simulink model "thermal_closed_loop_model"  (R2023a)
settings: Solver=ode23t  StartTime=0.0  StopTime=600  RelTol=1e-3
PostLoadFcn:
  | run('thermal_model_parameters.m')
  | run('thermal_harness_parameters.m')
  | run('thermal_variants_config.m')
values from neighbouring files (symbols this model uses):
  air_cp = 1004    [cathode_subsystem_parameters.m]    (also in thermal_subsystem_parameters.m)
  air_HC_min = 10    [cathode_subsystem_parameters.m]    (also in thermal_subsystem_parameters.m)
  air_HC_nom = 100    [cathode_subsystem_parameters.m]    (also in thermal_subsystem_parameters.m)
  air_rho = 1.2    [cathode_subsystem_parameters.m]    (also in thermal_subsystem_parameters.m)
  air_vel_nom = 1    [cathode_subsystem_parameters.m]    (also in thermal_subsystem_parameters.m)
  coolant_initial_pressure = 0.111325    [cathode_subsystem_parameters.m]    (also in thermal_subsystem_parameters.m)
  coolant_initial_temperature = 293.15    [cathode_subsystem_parameters.m]    (also in thermal_subsystem_parameters.m)
  coolant_tube_D = 0.05    [cathode_subsystem_parameters.m]    (also in thermal_subsystem_parameters.m)
  Hydrowell_VTS =     [Hydrowell_values_VLV.mat]
  radiator_area_air = 0.10260000000000001    (= 0.1026)    [cathode_subsystem_parameters.m]    (also in thermal_subsystem_parameters.m)
  radiator_area_fins = 2.5436250000000005    (= 2.543625)    [cathode_subsystem_parameters.m]    (also in thermal_subsystem_parameters.m)
  radiator_area_primary = 0.44452500000000011    (= 0.444525)    [cathode_subsystem_parameters.m]    (also in thermal_subsystem_parameters.m = 2 * radiator_tube_length * radiator_width * (radiator_fin_ro)
  radiator_n_tubes = 20    [cathode_subsystem_parameters.m]    (also in thermal_subsystem_parameters.m)
  radiator_tube_height = 0.0015    [cathode_subsystem_parameters.m]    (also in thermal_subsystem_parameters.m)
  radiator_tube_length = 0.45    [cathode_subsystem_parameters.m]    (also in thermal_subsystem_parameters.m)
  radiator_width = 0.025    [cathode_subsystem_parameters.m]    (also in thermal_subsystem_parameters.m)
  tcp_time_constant = 2    [cathode_subsystem_parameters.m]    (also in thermal_subsystem_parameters.m)
undefined symbols (not defined in the file or in its folder): sigbuilder_block, stack
libraries: fl_lib x153, nesl_utility x122, SimscapeFluids_lib x16, slpidlib x5, simulink x1
(part 2 of 8)

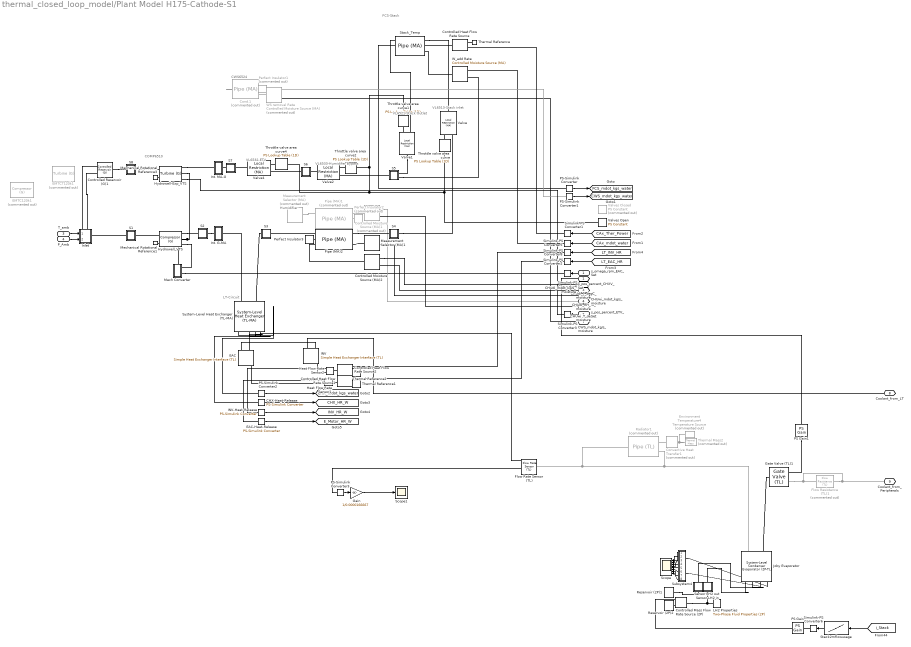
== system thermal_closed_loop_model/Plant Model H175-Cathode-S1 ==
  note: LT-Circuit
  note: Humidifier
  note: COMP6510
  note: FCS-Stack
  note: VL6513-Stack inlet
  note: VL6521-Stack Outlet
  note: VL6533-Humidifer Bypass
  note: CWS6524
  note: VL6532-ETV
  s_omega_rpm_EAC_Set : Inport
  s_pos_percent_ETV_Set : Inport  Port=2
  T_amb : Inport  Port=3
  P_Amb : Inport  Port=4
  CHX-Heat-Release : nesl_utility/PS-Simulink Converter  PhysicalDomain=network_engine_domain  SubClassName=ps_output  LeftPortType=input  RightPortType=output  PseudoPeriodic=off  Frequencies=[]  VectorFormat=inherit  Unit=inherit  AffineConversion=off
  Cond.1 : fl_lib/Moist Air/Elements/Pipe (MA)  Commented=on  length=1 m  area=1 m^2  Dh=.1 m  length_add=.1 m  roughness=15e-6 m  Re_lam=2000  Re_tur=4000  shape_factor=64  Nu_lam=3.66  wall_condensation=simscape.enum.onoff.on  RH_ws=.2  time_constant=1e-3 s  moisture_trace_gas_source=foundation.enum.moisture_trace_gas_source.controlled  moisture_source_spec=foundation.enum.moisture_source_spec.vapor  moisture_mass_flow=0 kg/s  moisture_temperature_spec=foundation.enum.temperature_spec.atmospheric  moisture_temperature=293.15 K  trace_gas_mass_flow=0 kg/s  trace_gas_temperature_spec=foundation.enum.temperature_spec.atmospheric  trace_gas_temperature=293.15 K  p_I_specify=off  p_I_priority=High  p_I=0.101325 MPa  p_I_nominal_specify=off  p_I_nominal_unit=MPa  p_I_nominal_value=1  T_I_specify=off  T_I_priority=High  T_I=293.15 K  T_I_nominal_specify=off  T_I_nominal_unit=K  T_I_nominal_value=1  RH_I_specify=off  RH_I_priority=High  RH_I=0  RH_I_nominal_specify=off  RH_I_nominal_unit=1  RH_I_nominal_value=1  x_w_I_specify=off  x_w_I_priority=None  x_w_I=0  x_w_I_nominal_specify=off  x_w_I_nominal_unit=1  x_w_I_nominal_value=1  y_w_I_specify=off  y_w_I_priority=None  y_w_I=0  y_w_I_nominal_specify=off  y_w_I_nominal_unit=1  y_w_I_nominal_value=1  HR_I_specify=off  HR_I_priority=None  HR_I=0  HR_I_nominal_specify=off  HR_I_nominal_unit=1  HR_I_nominal_value=1  x_g_I_specify=off  x_g_I_priority=High  x_g_I=0  x_g_I_nominal_specify=off  x_g_I_nominal_unit=1  x_g_I_nominal_value=1  y_g_I_specify=off  y_g_I_priority=None  y_g_I=0  y_g_I_nominal_specify=off  y_g_I_nominal_unit=1  y_g_I_nominal_value=1
      settings: InternalSimscapePortConfiguration="{\"Bottom\":[],\"Left\":[{\"id\":\"A\",\"label\":\"A\",\"type\":\"foundation.moist_air.moist_air\"},{\"id\":\"H\",\"label\":\"H\",\"type\":\"foundation.thermal.thermal\"},{\"id\":\"S\",\"label\":\"S\",\"type\":\"foundation.moist_air.moist_air_source\"}],\"Right\":[{\"id\":\"B\",\"label\":\"B\",\"type\":\"foundation.moist_air.moist_air\"},{\"id\":\"W\",\"label\":\"W\",\"type\":\"output\"},{\"id\":\"F\",\"label\":\"F\",\"type\":\"output\"}],\"Top\":[]}"
  Controlled Heat Flow Rate Source : fl_lib/Thermal/Thermal Sources/Controlled Heat Flow Rate Source
  Controlled Heat Flow Rate Source1 : fl_lib/Thermal/Thermal Sources/Controlled Heat Flow Rate Source
  Controlled Heat Flow Rate Source2 : fl_lib/Thermal/Thermal Sources/Controlled Heat Flow Rate Source
  Controlled Mass Flow Rate Source (2P) : fl_lib/Two-Phase Fluid/Sources/Controlled Mass Flow Rate Source (2P)  power_spec=foundation.enum.power_spec.none  area_A=.005^2*pi m^2  area_B=.005^2*pi m^2
      settings: InternalSimscapePortConfiguration="{\"Bottom\":[],\"Left\":[{\"id\":\"A\",\"label\":\"A\",\"type\":\"foundation.two_phase_fluid.two_phase_fluid\"},{\"id\":\"M\",\"label\":\"M\",\"type\":\"input\"}],\"Right\":[{\"id\":\"B\",\"label\":\"B\",\"type\":\"foundation.two_phase_fluid.two_phase_fluid\"}],\"Top\":[]}"
  Controlled Moisture Source (MA)1 : fl_lib/Moist Air/Sources/Moisture & Trace Gas Sources/Controlled Moisture Source (MA)  Commented=on  moisture_source_spec=foundation.enum.moisture_source_spec.vapor  Phi_S_specify=off  Phi_S_priority=None  Phi_S=0 kW  Phi_S_nominal_specify=off  Phi_S_nominal_unit=kW  Phi_S_nominal_value=1  mdot_w_S_specify=off  mdot_w_S_priority=None  mdot_w_S=0 kg/s  mdot_w_S_nominal_specify=off  mdot_w_S_nominal_unit=kg/s  mdot_w_S_nominal_value=1
      settings: InternalSimscapePortConfiguration="{\"Bottom\":[],\"Left\":[{\"id\":\"S\",\"label\":\"S\",\"type\":\"foundation.moist_air.moist_air_source\"}],\"Right\":[{\"id\":\"M\",\"label\":\"M\",\"type\":\"input\"},{\"id\":\"T\",\"label\":\"T\",\"type\":\"input\"}],\"Top\":[]}"
  Controlled Moisture Source (MA)2 : fl_lib/Moist Air/Sources/Moisture & Trace Gas Sources/Controlled Moisture Source (MA)  moisture_source_spec=foundation.enum.moisture_source_spec.vapor  Phi_S_specify=off  Phi_S_priority=None  Phi_S=0 kW  Phi_S_nominal_specify=off  Phi_S_nominal_unit=kW  Phi_S_nominal_value=1  mdot_w_S_specify=off  mdot_w_S_priority=None  mdot_w_S=0 kg/s  mdot_w_S_nominal_specify=off  mdot_w_S_nominal_unit=kg/s  mdot_w_S_nominal_value=1
      settings: InternalSimscapePortConfiguration="{\"Bottom\":[],\"Left\":[{\"id\":\"S\",\"label\":\"S\",\"type\":\"foundation.moist_air.moist_air_source\"}],\"Right\":[{\"id\":\"M\",\"label\":\"M\",\"type\":\"input\"},{\"id\":\"T\",\"label\":\"T\",\"type\":\"input\"}],\"Top\":[]}"
  Controlled Reservoir (G)1 : fl_lib/Gas/Elements/Controlled Reservoir (G)  area_A=0.002 m^2
      settings: InternalSimscapePortConfiguration="{\"Bottom\":[],\"Left\":[{\"id\":\"A\",\"label\":\"A\",\"type\":\"foundation.gas.gas\"}],\"Right\":[{\"id\":\"T_in\",\"label\":\"T\",\"type\":\"input\"},{\"id\":\"p_in\",\"label\":\"P\",\"type\":\"input\"}],\"Top\":[]}"
  Convective Heat Transfer1 : fl_lib/Thermal/Thermal Elements/Convective Heat Transfer  Commented=on  thermal_type=foundation.enum.constant_variable.constant  area=10.8 m^2  heat_tr_coeff=3465 W/(m^2 * K)  min_heat_tr_coeff=1e-3 W/(K*m^2)  T_specify=off  T_priority=None  T=0 K  T_nominal_specify=off  T_nominal_unit=K  T_nominal_value=1  Q_specify=off  Q_priority=None  Q=0 W  Q_nominal_specify=off  Q_nominal_unit=W  Q_nominal_value=1
  EAC : SimscapeFluids_lib/Fluid Network Interfaces/Heat Exchangers/Fundamental Components/Simple Heat Exchanger Interface (TL)  mdot_dp_TLU=[.3, .5, 1, 1.5, 2, 2.5] kg/s  p_diff_TLU=[3, 5, 10, 25, 35, 50] * 1e-3 MPa  T_ref_in=293.15 K  p_ref_in=0.101325 MPa  mdot_threshold=1e-3 kg/s  liquid_volume=0.01 m^3  area=0.01 m^2  dynamic_compressibility=simscape.enum.onoff.on  T0=293.15 K  p0=0.101325 MPa
      settings: InternalSimscapePortConfiguration="{\"Bottom\":[],\"Left\":[{\"id\":\"A\",\"label\":\"A\",\"type\":\"foundation.thermal_liquid.thermal_liquid\"},{\"id\":\"B\",\"label\":\"B\",\"type\":\"foundation.thermal_liquid.thermal_liquid\"}],\"Right\":[{\"id\":\"H\",\"label\":\"H\",\"type\":\"foundation.thermal.thermal\"},{\"id\":\"CP\",\"label\":\"CP\",\"type\":\"output\"},{\"id\":\"M\",\"label\":\"M\",\"type\":\"output\"}],\"Top\":[]}"
  EAC-Heat-Release : nesl_utility/PS-Simulink Converter  PhysicalDomain=network_engine_domain  SubClassName=ps_output  LeftPortType=input  RightPortType=output  PseudoPeriodic=off  Frequencies=[]  VectorFormat=inherit  Unit=inherit  AffineConversion=off
  EMTC120k1 : SimscapeFluids_lib/Gas/Turbomachinery/Compressor (G)  Commented=on  parameterization=fluids.gas.turbomachinery.enum.CompressorParameterization.Tabulated  NDes=10000 rpm  piDes=7.5  mdotDes=33 kg/s  efficiencyType=fluids.gas.turbomachinery.enum.EfficiencyType.Analytical  efficiencyValue=0.8  etaMax=0.887  etaMin=0.5  mdotMaxEff=30 kg/s  piMaxEff=7  omega_TLU=Fischer_EMTC120K_supplier_omega_TLU rpm  beta_TLU=Fischer_EMTC120K_supplier_beta_TLU  pr_TLU=Fischer_EMTC120K_supplier_pr_TLU  mdot_TLU=Fischer_EMTC120K_supplier_mdot_TLU g/s  eta_TLU=Fischer_EMTC120K_supplier_eta_TLU  SMFault=simscape.enum.assert.action.none  a=1.5  b=5  k=0.03  c=3  d=4  cCap=15  dCap=1.0  p_reference=0.101325 MPa  T_reference=288.15 K  mechanical_efficiency=0.98  area_A=.002 m^2  area_B=.002 m^2
      settings: LogSimulationData=on  InternalSimscapePortConfiguration="{\"Bottom\":[],\"Left\":[{\"id\":\"A\",\"label\":\"A\",\"type\":\"foundation.gas.gas\"},{\"id\":\"C\",\"label\":\"C\",\"type\":\"foundation.mechanical.rotational.rotational\"}],\"Right\":[{\"id\":\"B\",\"label\":\"B\",\"type\":\"foundation.gas.gas\"},{\"id\":\"R\",\"label\":\"R\",\"type\":\"foundation.mechanical.rotational.rotational\"},{\"id\":\"SM\",\"label\":\"SM\",\"type\":\"output\"}],\"Top\":[]}"
  EMTCT120k1 : SimscapeFluids_lib/Gas/Turbomachinery/Turbine (G)  Commented=on  parameterization=fluids.gas.turbomachinery.enum.TurbineParameterization.Tabulated1D  omega_TLU_2=[31000, 45000, 60000, 75000, 90000, 105000, 120000] rpm  variable_nozzle=true  min_nozzle_opening=1e-3  max_nozzle_opening=1  pr_nom=2  mdot_nom=0.08 kg/s  pr_mdot_TLU=[1.1667,1.405,1.791,2.18,2.5194]  mdot_TLU=[.0527,.08728,.1276,.1668,.1927] kg/s  pr_mdot_TLU_2=[1.217, 1.285, 1.323, 1.363, 1.402, 1.427, 1.495, 1.545, 1.6, 1.687, 1.747, 1.8074; 1.231, 1.302, 1.356, 1.404, 1.443, 1.473, 1.525, 1.577, 1.635, 1.709, 1.782, 1.845; 1.242, 1.328, 1.388, 1.437, 1.528, 1.617, 1.704, 1.811, 1.915, 1.979, 2.053, 2.1226; 1.244, 1.339, 1.417, 1.465, 1.528, 1.584, 1.692, 1.787, 1.899, 2, 2.075, 2.1492; 1.245, 1.34, 1.425, 1.492, 1.546, 1.684, 1.748, 1.882, 1.987, 2.084, 2.167, 2.2458; 1.251, 1.345, 1.442, 1.521, 1.596, 1.692, 1.849, 1.972, 2.1, 2.173, 2.259, 2.3424; 1.248, 1.348, 1.447, 1.516, 1.581, 1.651, 1.749, 1.839, 1.93, 2.024, 2.154, 2.242]  mdot_TLU_2=[40.403, 44.417, 46.653, 47.966, 48.97, 49.544, 50.001, 50.081, 50.086, 50.095, 50.09, 50.0922; 40.044, 43.754, 46.125, 47.626, 48.513, 49.105, 49.481, 49.58, 49.597, 49.624, 49.638, 49.633; 39.941, 43.795, 46.017, 47.335, 48.795, 49.199, 49.279, 49.27, 49.248, 49.23, 49.255, 49.2428; 39.896, 43.512, 45.914, 47.061, 48.011, 48.558, 48.943, 49.042, 49.069, 49.01, 49.046, 49.0266; 39.524, 42.934, 45.686, 46.743, 47.715, 48.67, 48.777, 48.836, 48.876, 48.836, 48.845, 48.8184; 39.439, 43.01, 45.556, 46.801, 47.792, 48.388, 48.634, 48.67, 48.639, 48.647, 48.625, 48.5912; 39.502, 42.849, 45.336, 46.385, 47.312, 47.877, 48.222, 48.397, 48.459, 48.482, 48.455, 48.414] kg/s  efficiency_constant=.954  pr_eta_TLU=[1.1667,1.405,1.791,2.18,2.5194]  eta_TLU=[0.6804,.76609,.7634,.7426,.72]  pr_eta_TLU_2=[1.224, 1.246, 1.292, 1.387, 1.457, 1.534, 1.61, 1.686, 1.743, 1.79, 1.871, 1.914; 1.237, 1.25, 1.28, 1.369, 1.459, 1.553, 1.629, 1.716, 1.799, 1.846, 1.927, 1.97; 1.241, 1.255, 1.283, 1.326, 1.401, 1.509, 1.591, 1.704, 1.806, 1.913, 1.994, 2.037; 1.25, 1.265, 1.308, 1.364, 1.456, 1.532, 1.637, 1.739, 1.851, 1.934, 2.042, 2.085; 1.281, 1.314, 1.371, 1.425, 1.498, 1.574, 1.647, 1.749, 1.878, 1.979, 2.091, 2.18; 1.252, 1.328, 1.425, 1.544, 1.642, 1.757, 1.873, 2.005, 2.1, 2.204, 2.248, 2.28; 1.382, 1.43, 1.495, 1.586, 1.688, 1.791, 1.887, 1.99, 2.079, 2.158, 2.249, 2.36]  eta_TLU_2=[.72, .754, .759, .739, .714, .679, .643, .603, .554, .524, .494, .48; .716, .757, .794, .819, .812, .788, .761, .728, .692, .662, .632, .618; .629, .691, .775, .831, .858, .869, .859, .842, .816, .782, .752, .738; .594, .668, .757, .804, .857, .883, .892, .893, .884, .865, .835, .821; .664, .72, .779, .823, .858, .883, .897, .905, .904, .896, .883, .868; .559, .61, .673, .741, .788, .835, .869, .895, .908, .899, .854, .751; .718, .785, .824, .855, .882, .9, .908, .906, .884, .857, .804, .701]  p_reference=1.6 bar  T_reference=85 degC  mechanical_efficiency=0.98  area_A=0.002 m^2  area_B=0.002 m^2
      settings: LogSimulationData=on  InternalSimscapePortConfiguration="{\"Bottom\":[],\"Left\":[{\"id\":\"A\",\"label\":\"A\",\"type\":\"foundation.gas.gas\"},{\"id\":\"R\",\"label\":\"R\",\"type\":\"foundation.mechanical.rotational.rotational\"},{\"id\":\"VN\",\"label\":\"VN\",\"type\":\"input\"}],\"Right\":[{\"id\":\"B\",\"label\":\"B\",\"type\":\"foundation.gas.gas\"},{\"id\":\"C\",\"label\":\"C\",\"type\":\"foundation.mechanical.rotational.rotational\"}],\"Top\":[]}"
  Environment Temperature4 : fl_lib/Thermal/Thermal Sources/Temperature Source  Commented=on  temperature=20 degC
  Flow Rate Sensor (TL) : fl_lib/Thermal Liquid/Sensors/Flow Rate Sensor (TL)  mass_flow_measure=true  volumetric_flow_measure=true  energy_flow_measure=true
      settings: InternalSimscapePortConfiguration="{\"Bottom\":[{\"id\":\"PHI\",\"label\":\"φ\",\"type\":\"output\"}],\"Left\":[{\"id\":\"A\",\"label\":\"A\",\"type\":\"foundation.thermal_liquid.thermal_liquid\"}],\"Right\":[{\"id\":\"B\",\"label\":\"B\",\"type\":\"foundation.thermal_liquid.thermal_liquid\"},{\"id\":\"M\",\"label\":\"M\",\"type\":\"output\"},{\"id\":\"V\",\"label\":\"V\",\"type\":\"output\"}],\"Top\":[]}"
  Flow Resistance (TL)1 : fl_lib/Thermal Liquid/Elements/Flow Resistance (TL)  Commented=on  delta_p_nominal=.05 bar  mdot_nominal=0.1665 kg/s  area=5.0670747909749775143163975128915e-4 m^2  laminar_fraction=1e-3
  Gain : Gain  Gain=1/0.0000166667
  Gate Valve (TL)1 : SimscapeFluids_lib/Thermal Liquid/Valves & Orifices/Flow Control Valves/Gate Valve (TL)  diam_orifice=.018/2.5 m  S_min=0 m  area_leak=1e-12 m^2  smoothing_factor=0.01  area=(.018/2)^2*pi m^2  Cd=0.7  Re_c=12
      settings: InternalSimscapePortConfiguration="{\"Bottom\":[],\"Left\":[{\"id\":\"A\",\"label\":\"A\",\"type\":\"foundation.thermal_liquid.thermal_liquid\"},{\"id\":\"S\",\"label\":\"S\",\"type\":\"input\"}],\"Right\":[{\"id\":\"B\",\"label\":\"B\",\"type\":\"foundation.thermal_liquid.thermal_liquid\"}],\"Top\":[]}"
  Heat Flow Rate Sensor1 : fl_lib/Thermal/Thermal Sensors/Heat Flow Rate Sensor
  Heat Flow Rate Sensor2 : fl_lib/Thermal/Thermal Sensors/Heat Flow Rate Sensor
  Hydrowell-Exp_VTS : SimscapeFluids_lib/Gas/Turbomachinery/Turbine (G)  parameterization=fluids.gas.turbomachinery.enum.TurbineParameterization.Tabulated1D  omega_TLU_2=[31000, 45000, 60000, 75000, 90000, 105000, 120000] rpm  variable_nozzle=true  min_nozzle_opening=1e-5  max_nozzle_opening=1  pr_nom=2  mdot_nom=0.08 kg/s  pr_mdot_TLU=Hydrowell_VTS.pr_expander*2  mdot_TLU=Hydrowell_VTS.mdot_expander*2 kg/s  pr_mdot_TLU_2=[1.217, 1.285, 1.323, 1.363, 1.402, 1.427, 1.495, 1.545, 1.6, 1.687, 1.747, 1.8074; 1.231, 1.302, 1.356, 1.404, 1.443, 1.473, 1.525, 1.577, 1.635, 1.709, 1.782, 1.845; 1.242, 1.328, 1.388, 1.437, 1.528, 1.617, 1.704, 1.811, 1.915, 1.979, 2.053, 2.1226; 1.244, 1.339, 1.417, 1.465, 1.528, 1.584, 1.692, 1.787, 1.899, 2, 2.075, 2.1492; 1.245, 1.34, 1.425, 1.492, 1.546, 1.684, 1.748, 1.882, 1.987, 2.084, 2.167, 2.2458; 1.251, 1.345, 1.442, 1.521, 1.596, 1.692, 1.849, 1.972, 2.1, 2.173, 2.259, 2.3424; 1.248, 1.348, 1.447, 1.516, 1.581, 1.651, 1.749, 1.839, 1.93, 2.024, 2.154, 2.242]*2  mdot_TLU_2=[40.403, 44.417, 46.653, 47.966, 48.97, 49.544, 50.001, 50.081, 50.086, 50.095, 50.09, 50.0922; 40.044, 43.754, 46.125, 47.626, 48.513, 49.105, 49.481, 49.58, 49.597, 49.624, 49.638, 49.633; 39.941, 43.795, 46.017, 47.335, 48.795, 49.199, 49.279, 49.27, 49.248, 49.23, 49.255, 49.2428; 39.896, 43.512, 45.914, 47.061, 48.011, 48.558, 48.943, 49.042, 49.069, 49.01, 49.046, 49.0266; 39.524, 42.934, 45.686, 46.743, 47.715, 48.67, 48.777, 48.836, 48.876, 48.836, 48.845, 48.8184; 39.439, 43.01, 45.556, 46.801, 47.792, 48.388, 48.634, 48.67, 48.639, 48.647, 48.625, 48.5912; 39.502, 42.849, 45.336, 46.385, 47.312, 47.877, 48.222, 48.397, 48.459, 48.482, 48.455, 48.414]*4 g/s  efficiency_constant=.954  pr_eta_TLU=Hydrowell_VTS.pr_expander*2  eta_TLU=Hydrowell_VTS.eta_expander  pr_eta_TLU_2=[1.224, 1.246, 1.292, 1.387, 1.457, 1.534, 1.61, 1.686, 1.743, 1.79, 1.871, 1.914; 1.237, 1.25, 1.28, 1.369, 1.459, 1.553, 1.629, 1.716, 1.799, 1.846, 1.927, 1.97; 1.241, 1.255, 1.283, 1.326, 1.401, 1.509, 1.591, 1.704, 1.806, 1.913, 1.994, 2.037; 1.25, 1.265, 1.308, 1.364, 1.456, 1.532, 1.637, 1.739, 1.851, 1.934, 2.042, 2.085; 1.281, 1.314, 1.371, 1.425, 1.498, 1.574, 1.647, 1.749, 1.878, 1.979, 2.091, 2.18; 1.252, 1.328, 1.425, 1.544, 1.642, 1.757, 1.873, 2.005, 2.1, 2.204, 2.248, 2.28; 1.382, 1.43, 1.495, 1.586, 1.688, 1.791, 1.887, 1.99, 2.079, 2.158, 2.249, 2.36]  eta_TLU_2=[.72, .754, .759, .739, .714, .679, .643, .603, .554, .524, .494, .48; .716, .757, .794, .819, .812, .788, .761, .728, .692, .662, .632, .618; .629, .691, .775, .831, .858, .869, .859, .842, .816, .782, .752, .738; .594, .668, .757, .804, .857, .883, .892, .893, .884, .865, .835, .821; .664, .72, .779, .823, .858, .883, .897, .905, .904, .896, .883, .868; .559, .61, .673, .741, .788, .835, .869, .895, .908, .899, .854, .751; .718, .785, .824, .855, .882, .9, .908, .906, .884, .857, .804, .701]  p_reference=1.015 bar  T_reference=293 K  mechanical_efficiency=0.98  area_A=0.002 m^2  area_B=0.002 m^2
      settings: LogSimulationData=on  InternalSimscapePortConfiguration="{\"Bottom\":[],\"Left\":[{\"id\":\"A\",\"label\":\"A\",\"type\":\"foundation.gas.gas\"},{\"id\":\"R\",\"label\":\"R\",\"type\":\"foundation.mechanical.rotational.rotational\"},{\"id\":\"VN\",\"label\":\"VN\",\"type\":\"input\"}],\"Right\":[{\"id\":\"B\",\"label\":\"B\",\"type\":\"foundation.gas.gas\"},{\"id\":\"C\",\"label\":\"C\",\"type\":\"foundation.mechanical.rotational.rotational\"}],\"Top\":[]}"
  Hydrowell_VTS : SimscapeFluids_lib/Gas/Turbomachinery/Compressor (G)  parameterization=fluids.gas.turbomachinery.enum.CompressorParameterization.Tabulated  NDes=10000 rpm  piDes=7.5  mdotDes=33 kg/s  efficiencyType=fluids.gas.turbomachinery.enum.EfficiencyType.Analytical  efficiencyValue=0.8  etaMax=0.887  etaMin=0.5  mdotMaxEff=30 kg/s  piMaxEff=7  omega_TLU=Hydrowell_VTS.omega rpm  beta_TLU=Hydrowell_VTS.beta  pr_TLU=Hydrowell_VTS.pr*2  mdot_TLU=Hydrowell_VTS.mdot*2 g/s  eta_TLU=Hydrowell_VTS.eta  SMFault=simscape.enum.assert.action.none  a=1.5  b=5  k=0.03  c=3  d=4  cCap=15  dCap=1.0  p_reference=0.101325 MPa  T_reference=288.15 K  mechanical_efficiency=0.98  area_A=.002 m^2  area_B=.002 m^2
      settings: LogSimulationData=on  InternalSimscapePortConfiguration="{\"Bottom\":[],\"Left\":[{\"id\":\"A\",\"label\":\"A\",\"type\":\"foundation.gas.gas\"},{\"id\":\"C\",\"label\":\"C\",\"type\":\"foundation.mechanical.rotational.rotational\"}],\"Right\":[{\"id\":\"B\",\"label\":\"B\",\"type\":\"foundation.gas.gas\"},{\"id\":\"R\",\"label\":\"R\",\"type\":\"foundation.mechanical.rotational.rotational\"},{\"id\":\"SM\",\"label\":\"SM\",\"type\":\"output\"}],\"Top\":[]}"
  INV : SimscapeFluids_lib/Fluid Network Interfaces/Heat Exchangers/Fundamental Components/Simple Heat Exchanger Interface (TL)  mdot_dp_TLU=[.3, .5, 1, 1.5, 2, 2.5] kg/s  p_diff_TLU=[3, 5, 10, 25, 35, 50] * 1e-3 MPa  T_ref_in=293.15 K  p_ref_in=0.101325 MPa  mdot_threshold=1e-3 kg/s  liquid_volume=0.01 m^3  area=0.01 m^2  dynamic_compressibility=simscape.enum.onoff.on  T0=293.15 K  p0=0.101325 MPa
      settings: InternalSimscapePortConfiguration="{\"Bottom\":[],\"Left\":[{\"id\":\"A\",\"label\":\"A\",\"type\":\"foundation.thermal_liquid.thermal_liquid\"},{\"id\":\"B\",\"label\":\"B\",\"type\":\"foundation.thermal_liquid.thermal_liquid\"}],\"Right\":[{\"id\":\"H\",\"label\":\"H\",\"type\":\"foundation.thermal.thermal\"},{\"id\":\"CP\",\"label\":\"CP\",\"type\":\"output\"},{\"id\":\"M\",\"label\":\"M\",\"type\":\"output\"}],\"Top\":[]}"
  INV-Heat-Release : nesl_utility/PS-Simulink Converter  PhysicalDomain=network_engine_domain  SubClassName=ps_output  LeftPortType=input  RightPortType=output  PseudoPeriodic=off  Frequencies=[]  VectorFormat=inherit  Unit=inherit  AffineConversion=off
  Inlet : Subsystem
      settings: PortSchema="{\"entries\":[{\"content\":{\"sides\":[{\"content\":{\"connectorIds\":[\"In1\",\"In2\"]},\"type\":\"ConnectorPlacement.EquallySpacedRectSide\",\"uuid\":\"383c8b90-d22b-483c-be09-d78d9bde0881\"},{\"content\":{\"connectorIds\":[\"RConn1\"],\"side\":\"RIGHT\"},\"type\":\"ConnectorPlacement.EquallySpacedRectSide\",\"uuid\":\"3dc3e004-4331-4c40-8051-329aa9250422\"},{\"content\":{\"connectorIds\":[\"LConn1\",\"LConn2\"],\"side\":\"TOP\"},\"type\":\"ConnectorPlacement.EquallySpacedRectSide\",\"uuid\":\"aff35d8f-ac03-451a-b72e-dc7bd89924e8\"},{\"content\":{\"side\":\"BOTTOM\"},\"type\":\"ConnectorPlacement.EquallySpacedRectSide\",\"uuid\":\"82493911-a5c4-468a-a003-983b92ffd105\"}]},\"type\":\"ConnectorPlacement.EquallySpacedConnector\",\"uuid\":\"d9a1e9aa-22f5-4e42-bf15-8a8ecd9f58f9\"}],\"packageUris\":[\"http://schema.mathworks.com/mf0/Connector/R2020b\"],\"version\":\"1.0\"}"
  Int. G-MA : Subsystem
  Int. MA-G : Subsystem
  Joby Evaporator : SimscapeFluids_lib/Fluid Network Interfaces/Heat Exchangers/System-Level Condenser Evaporator (2P-TL)  flow_arrangement=fluids.interfaces.heat_exchangers.enum.SystemLevelFlowArrangement2PTL.Counter  wall_thermal_mass=simscape.enum.onoff.off  mass_wall=1 kg  cp_wall=490 J/(K*kg)  area_A1=.005^2*pi m^2  area_B1=.005^2*pi m^2  area_A2=4.90874e-4 m^2  area_B2=4.90874e-4 m^2  operating_condition_2P=fluids.interfaces.heat_exchangers.enum.SystemLevelOperatingCondition2PTL.Evaporator  mdot_nominal_2P=.002 kg/s  delta_p_nominal_2P=.03 bar  pressure_spec_cond_2P=fluids.interfaces.heat_exchangers.enum.SystemLevelPressureSpecCondenser2P.InletPressure  pressure_spec_evap_2P=fluids.interfaces.heat_exchangers.enum.SystemLevelPressureSpecEvaporator2P.InletPressure  p_in_nominal_2P=5 bar  T_cond_nominal_2P=313.15 K  T_evap_nominal_2P=243.15 K  inlet_spec_2P=fluids.interfaces.heat_exchangers.enum.SystemLevelInletSpec2P.Temperature  T_in_nominal_2P=23 K  h_in_nominal_2P=87 kJ/kg  x_in_nominal_2P=1  capacity_spec_2P=fluids.interfaces.heat_exchangers.enum.SystemLevelCapacitySpec.HeatTransfer  Q_nominal=8 kW  outlet_spec_cond_2P=fluids.interfaces.heat_exchangers.enum.SystemLevelOutletSpecCondenser2P.Enthalpy  outlet_spec_evap_2P=fluids.interfaces.heat_exchangers.enum.SystemLevelOutletSpecEvaporator2P.Enthalpy  delta_T_sub_nominal_2P=5 deltaK  delta_T_sup_nominal_2P=1 deltaK  h_out_nominal_2P=4200 kJ/kg  x_out_nominal_2P=1  volume_2P=.002 l  init_spec_2P=fluids.interfaces.heat_exchangers.enum.SystemLevelInitialConditionSpec.Operating  energy_spec_2P=foundation.enum.energy_spec.enthalpy  p_init_2P=5 bar  T_init_2P=293.15 K  x_init_2P=0.5  alpha_init_2P=0.5  h_init_2P=-41.06 kJ/kg  u_init_2P=1500 kJ/kg  mdot_nominal_TL=1 kg/s  delta_p_nominal_TL=0.01 bar  p_in_nominal_TL=1.3 bar  T_in_nominal_TL=273.15+25 K  volume_TL=.5 l  init_spec_TL=fluids.interfaces.heat_exchangers.enum.SystemLevelInitialConditionSpec.Operating  p_init_TL=0.101325 MPa  T_init_TL=293.15 K  a_liq_2P=0.023  a_mix_2P=0.005  a_vap_2P=0.023  b_2P=0.8  c_2P=0.33  a_TL=0.023  b_TL=0.8  c_TL=0.33
      settings: LogSimulationData=on  InternalSimscapePortConfiguration="{\"Bottom\":[],\"Left\":[{\"id\":\"A1\",\"label\":\"A1\",\"type\":\"foundation.two_phase_fluid.two_phase_fluid\"},{\"id\":\"B1\",\"label\":\"B1\",\"type\":\"foundation.two_phase_fluid.two_phase_fluid\"}],\"Right\":[{\"id\":\"A2\",\"label\":\"A2\",\"type\":\"foundation.thermal_liquid.thermal_liquid\"},{\"id\":\"B2\",\"label\":\"B2\",\"type\":\"foundation.thermal_liquid.thermal_liquid\"}],\"Top\":[{\"id\":\"Q1\",\"label\":\"Q1\",\"type\":\"output\"},{\"id\":\"Q2\",\"label\":\"Q2\",\"type\":\"output\"}]}"
  LH2 Properties : fl_lib/Two-Phase Fluid/Utilities/Two-Phase Fluid Properties (2P)  u_min=H2PropertyTables.u_min kJ/kg  u_max=H2PropertyTables.u_max kJ/kg  p_TLU=H2PropertyTables.p bar  p_crit=H2PropertyTables.p_crit bar  critical_region=foundation.enum.critical_region.no_clip  p_crit_fraction=0.12  p_atm=0.101325 MPa  properties_range_check=simscape.enum.assert.action.none  q_rev=0.01 Pa  unorm_liq=H2PropertyTables.liquid.unorm  v_liq=H2PropertyTables.liquid.v m^3/kg  s_liq=H2PropertyTables.liquid.s kJ/(kg*K)  T_liq=H2PropertyTables.liquid.T K  nu_liq=H2PropertyTables.liquid.nu mm^2/s  k_liq=H2PropertyTables.liquid.k W/(m*K)  Pr_liq=H2PropertyTables.liquid.Pr  u_sat_liq=H2PropertyTables.liquid.u_sat kJ/kg  unorm_vap=H2PropertyTables.vapor.unorm  v_vap=H2PropertyTables.vapor.v m^3/kg  s_vap=H2PropertyTables.vapor.s kJ/(kg*K)  T_vap=H2PropertyTables.vapor.T K  nu_vap=H2PropertyTables.vapor.nu mm^2/s  k_vap=H2PropertyTables.vapor.k W/(m*K)  Pr_vap=H2PropertyTables.vapor.Pr  u_sat_vap=H2PropertyTables.vapor.u_sat kJ/kg
      settings: InternalSimscapePortConfiguration="{\"Bottom\":[],\"Left\":[],\"Right\":[{\"id\":\"A\",\"label\":\"\",\"type\":\"foundation.two_phase_fluid.two_phase_fluid\"}],\"Top\":[]}"
  Measurement Selector (MA) : fl_lib/Moist Air/Sensors/Measurement Selector (MA)  Commented=on  moisture_spec=foundation.enum.moisture_spec.relative_humidity  trace_gas_spec=foundation.enum.trace_gas_spec.mole_fraction
  Measurement Selector (MA)1 : fl_lib/Moist Air/Sensors/Measurement Selector (MA)  moisture_spec=foundation.enum.moisture_spec.relative_humidity  trace_gas_spec=foundation.enum.trace_gas_spec.mole_fraction
  Mech Converter : Subsystem
      settings: PortSchema="{\"entries\":[{\"content\":{\"sides\":[{\"content\":{},\"type\":\"ConnectorPlacement.EquallySpacedRectSide\",\"uuid\":\"f204080c-20ff-4b02-9705-6e1b54158713\"},{\"content\":{\"connectorIds\":[\"RConn1\",\"RConn2\"],\"side\":\"RIGHT\"},\"type\":\"ConnectorPlacement.EquallySpacedRectSide\",\"uuid\":\"3afd75cf-16d9-416a-a176-5f277eec2a64\"},{\"content\":{\"connectorIds\":[\"LConn1\"],\"side\":\"TOP\"},\"type\":\"ConnectorPlacement.EquallySpacedRectSide\",\"uuid\":\"c26ef975-7cc2-47e8-a2f6-f206167626c7\"}]},\"type\":\"ConnectorPlacement.EquallySpacedConnector\",\"uuid\":\"b56aa784-ee28-43ca-98b1-bf8a16682298\"}],\"packageUris\":[\"http://schema.mathworks.com/mf0/Connector/R2020b\"],\"version\":\"1.0\"}"
  Mechanical Rotational Reference1 : fl_lib/Mechanical/Rotational Elements/Mechanical Rotational Reference
  Mechanical Rotational Reference3 : fl_lib/Mechanical/Rotational Elements/Mechanical Rotational Reference
  PS Gain : fl_lib/Physical Signals/Functions/PS Gain  gain=.001
  PS Gain1 : fl_lib/Physical Signals/Functions/PS Gain  gain=0.5
  PS-Simulink Converter{,1..3} (4 alike) : nesl_utility/PS-Simulink Converter  PhysicalDomain=network_engine_domain  SubClassName=ps_output  LeftPortType=input  RightPortType=output  PseudoPeriodic=off  Frequencies=[]  VectorFormat=inherit  Unit=inherit  AffineConversion=off
  Perfect Insulator1 : fl_lib/Thermal/Thermal Elements/Perfect Insulator  Commented=on  T_specify=off  T_priority=None  T=293.15 K  T_nominal_specify=off  T_nominal_unit=K  T_nominal_value=1
  Perfect Insulator2 : fl_lib/Thermal/Thermal Elements/Perfect Insulator  Commented=on  T_specify=off  T_priority=None  T=0 K  T_nominal_specify=off  T_nominal_unit=K  T_nominal_value=1
  Perfect Insulator3 : fl_lib/Thermal/Thermal Elements/Perfect Insulator  T_specify=off  T_priority=None  T=0 K  T_nominal_specify=off  T_nominal_unit=K  T_nominal_value=1
  Pipe (MA)1 : fl_lib/Moist Air/Elements/Pipe (MA)  Commented=on  length=0.25 m  area=pi*0.05^2/4 m^2  Dh=0.05 m  length_add=0.1 m  roughness=15e-6 m  Re_lam=2000  Re_tur=4000  shape_factor=64  Nu_lam=3.66  wall_condensation=simscape.enum.onoff.off  RH_ws=1  time_constant=1e-3 s  moisture_trace_gas_source=foundation.enum.moisture_trace_gas_source.controlled  moisture_source_spec=foundation.enum.moisture_source_spec.vapor  moisture_mass_flow=0 kg/s  moisture_temperature_spec=foundation.enum.temperature_spec.atmospheric  moisture_temperature=293.15 K  trace_gas_mass_flow=0 kg/s  trace_gas_temperature_spec=foundation.enum.temperature_spec.atmospheric  trace_gas_temperature=293.15 K  p_I_specify=off  p_I_priority=High  p_I=env_p MPa  p_I_nominal_specify=off  p_I_nominal_unit=MPa  p_I_nominal_value=1  T_I_specify=off  T_I_priority=High  T_I=env_T degC  T_I_nominal_specify=off  T_I_nominal_unit=K  T_I_nominal_value=1  RH_I_specify=off  RH_I_priority=High  RH_I=env_RH  RH_I_nominal_specify=off  RH_I_nominal_unit=1  RH_I_nominal_value=1  x_w_I_specify=off  x_w_I_priority=None  x_w_I=0  x_w_I_nominal_specify=off  x_w_I_nominal_unit=1  x_w_I_nominal_value=1  y_w_I_specify=off  y_w_I_priority=None  y_w_I=0  y_w_I_nominal_specify=off  y_w_I_nominal_unit=1  y_w_I_nominal_value=1  HR_I_specify=off  HR_I_priority=None  HR_I=0  HR_I_nominal_specify=off  HR_I_nominal_unit=1  HR_I_nominal_value=1  x_g_I_specify=off  x_g_I_priority=None  x_g_I=0  x_g_I_nominal_specify=off  x_g_I_nominal_unit=1  x_g_I_nominal_value=1  y_g_I_specify=off  y_g_I_priority=High  y_g_I=env_yO2  y_g_I_nominal_specify=off  y_g_I_nominal_unit=1  y_g_I_nominal_value=1
      settings: InternalSimscapePortConfiguration="{\"Bottom\":[],\"Left\":[{\"id\":\"A\",\"label\":\"A\",\"type\":\"foundation.moist_air.moist_air\"},{\"id\":\"H\",\"label\":\"H\",\"type\":\"foundation.thermal.thermal\"},{\"id\":\"S\",\"label\":\"S\",\"type\":\"foundation.moist_air.moist_air_source\"}],\"Right\":[{\"id\":\"B\",\"label\":\"B\",\"type\":\"foundation.moist_air.moist_air\"},{\"id\":\"W\",\"label\":\"W\",\"type\":\"output\"},{\"id\":\"F\",\"label\":\"F\",\"type\":\"output\"}],\"Top\":[]}"
  Pipe (MA)2 : fl_lib/Moist Air/Elements/Pipe (MA)  length=0.25 m  area=pi*0.05^2/4 m^2  Dh=0.05 m  length_add=0.1 m  roughness=15e-6 m  Re_lam=2000  Re_tur=4000  shape_factor=64  Nu_lam=3.66  wall_condensation=simscape.enum.onoff.off  RH_ws=1  time_constant=1e-3 s  moisture_trace_gas_source=foundation.enum.moisture_trace_gas_source.controlled  moisture_source_spec=foundation.enum.moisture_source_spec.vapor  moisture_mass_flow=0 kg/s  moisture_temperature_spec=foundation.enum.temperature_spec.atmospheric  moisture_temperature=293.15 K  trace_gas_mass_flow=0 kg/s  trace_gas_temperature_spec=foundation.enum.temperature_spec.atmospheric  trace_gas_temperature=293.15 K  p_I_specify=off  p_I_priority=High  p_I=env_p MPa  p_I_nominal_specify=off  p_I_nominal_unit=MPa  p_I_nominal_value=1  T_I_specify=off  T_I_priority=High  T_I=20 degC  T_I_nominal_specify=off  T_I_nominal_unit=K  T_I_nominal_value=1  RH_I_specify=off  RH_I_priority=High  RH_I=0.5  RH_I_nominal_specify=off  RH_I_nominal_unit=1  RH_I_nominal_value=1  x_w_I_specify=off  x_w_I_priority=None  x_w_I=0  x_w_I_nominal_specify=off  x_w_I_nominal_unit=1  x_w_I_nominal_value=1  y_w_I_specify=off  y_w_I_priority=None  y_w_I=0  y_w_I_nominal_specify=off  y_w_I_nominal_unit=1  y_w_I_nominal_value=1  HR_I_specify=off  HR_I_priority=None  HR_I=0  HR_I_nominal_specify=off  HR_I_nominal_unit=1  HR_I_nominal_value=1  x_g_I_specify=off  x_g_I_priority=None  x_g_I=0  x_g_I_nominal_specify=off  x_g_I_nominal_unit=1  x_g_I_nominal_value=1  y_g_I_specify=off  y_g_I_priority=High  y_g_I=env_yO2  y_g_I_nominal_specify=off  y_g_I_nominal_unit=1  y_g_I_nominal_value=1
      settings: InternalSimscapePortConfiguration="{\"Bottom\":[],\"Left\":[{\"id\":\"A\",\"label\":\"A\",\"type\":\"foundation.moist_air.moist_air\"},{\"id\":\"H\",\"label\":\"H\",\"type\":\"foundation.thermal.thermal\"},{\"id\":\"S\",\"label\":\"S\",\"type\":\"foundation.moist_air.moist_air_source\"}],\"Right\":[{\"id\":\"B\",\"label\":\"B\",\"type\":\"foundation.moist_air.moist_air\"},{\"id\":\"W\",\"label\":\"W\",\"type\":\"output\"},{\"id\":\"F\",\"label\":\"F\",\"type\":\"output\"}],\"Top\":[]}"
  Radiator1 : fl_lib/Thermal Liquid/Elements/Pipe (TL)  Commented=on  length=1 m  area=10.8 m^2  Dh=.25 m  length_add=1 m  roughness=15e-6 m  Re_lam=2000  Re_tur=4000  shape_factor=64  Nu_lam=500  dynamic_compressibility=simscape.enum.onoff.on  inertia=simscape.enum.onoff.off  p0=.103 MPa  T0=20 degC  mdot0=0 kg/s
  Reservoir (2P)1 : fl_lib/Two-Phase Fluid/Elements/Reservoir (2P)  pressure_spec=foundation.enum.pressure_spec.specified  reservoir_pressure=5 bar  reservoir_condensing_temperature=373.15 K  reservoir_evaporating_temperature=373.15 K  energy_spec=foundation.enum.ReservoirEnergySpec2P.Quality  reservoir_temperature=293.15 K  reservoir_quality=0.95  reservoir_void_fraction=0.5  reservoir_enthalpy=1500 kJ/kg  reservoir_internal_energy=1500 kJ/kg  reservoir_subcooling=5 deltaK  reservoir_superheating=5 deltaK  area_A=.002 m^2
  Reservoir (2P)2 : fl_lib/Two-Phase Fluid/Elements/Reservoir (2P)  pressure_spec=foundation.enum.pressure_spec.specified  reservoir_pressure=5 bar  reservoir_condensing_temperature=373.15 K  reservoir_evaporating_temperature=373.15 K  energy_spec=foundation.enum.ReservoirEnergySpec2P.Temperature  reservoir_temperature=26 K  reservoir_quality=0.95  reservoir_void_fraction=0.5  reservoir_enthalpy=1500 kJ/kg  reservoir_internal_energy=1500 kJ/kg  reservoir_subcooling=5 deltaK  reservoir_superheating=5 deltaK  area_A=.005^2*pi m^2
  S1 : Subsystem
  S2 : Subsystem
  S3 : Subsystem
  S4 : Subsystem
  S5 : Subsystem
  S6 : Subsystem
  S7 : Subsystem
  S8 : Subsystem
  Scope : Scope  NumInputPorts=8
  Scope1 : Scope
  Sensor LH2 in : Subsystem
      mask Display: disp('\Phi', 'texmode', 'on')
  Sensor LH2 out : Subsystem
      mask Display: disp('\Phi', 'texmode', 'on')
  Simulink-PS Converter{1..6,8} (7 alike) : nesl_utility/Simulink-PS Converter  PhysicalDomain=network_engine_domain  SubClassName=ps_input  LeftPortType=input  RightPortType=output  PseudoPeriodic=off  Frequencies=[]  NoiseDistribution=none  NoiseParameters=[]  Unit=1  AffineConversion=off  FilteringAndDerivatives=provide  SimscapeFilterOrder=1  InputFilterTimeConstant=0.001  UdotUserProvided=0
  Stack2mflowusage : Lookup_n-D  NumberOfTableDimensions=1  BreakpointsForDimension1=[0:50:400]  Table=|  InternalRulePriority=Speed  RndMeth=Simplest
      | [0.025,
      | 0.32,
      | 0.63,
      | 0.92,
      | 1.18,
      | 1.52,
      | 1.80,
      | 2.09,
      | 2.39]
  Stack_Temp : fl_lib/Moist Air/Elements/Pipe (MA)  length=1 m  area=1 m^2  Dh=.2 m  length_add=.1 m  roughness=15e-6 m  Re_lam=2000  Re_tur=4000  shape_factor=64  Nu_lam=3.66  wall_condensation=simscape.enum.onoff.off  RH_ws=1  time_constant=1e-3 s  moisture_trace_gas_source=foundation.enum.moisture_trace_gas_source.controlled  moisture_source_spec=foundation.enum.moisture_source_spec.vapor  moisture_mass_flow=0 kg/s  moisture_temperature_spec=foundation.enum.temperature_spec.atmospheric  moisture_temperature=293.15 K  trace_gas_mass_flow=0 kg/s  trace_gas_temperature_spec=foundation.enum.temperature_spec.atmospheric  trace_gas_temperature=293.15 K  p_I_specify=off  p_I_priority=High  p_I=0.101325 MPa  p_I_nominal_specify=off  p_I_nominal_unit=MPa  p_I_nominal_value=1  T_I_specify=off  T_I_priority=High  T_I=293.15 K  T_I_nominal_specify=off  T_I_nominal_unit=K  T_I_nominal_value=1  RH_I_specify=off  RH_I_priority=High  RH_I=0  RH_I_nominal_specify=off  RH_I_nominal_unit=1  RH_I_nominal_value=1  x_w_I_specify=off  x_w_I_priority=None  x_w_I=0  x_w_I_nominal_specify=off  x_w_I_nominal_unit=1  x_w_I_nominal_value=1  y_w_I_specify=off  y_w_I_priority=None  y_w_I=0  y_w_I_nominal_specify=off  y_w_I_nominal_unit=1  y_w_I_nominal_value=1  HR_I_specify=off  HR_I_priority=None  HR_I=0  HR_I_nominal_specify=off  HR_I_nominal_unit=1  HR_I_nominal_value=1  x_g_I_specify=off  x_g_I_priority=High  x_g_I=0  x_g_I_nominal_specify=off  x_g_I_nominal_unit=1  x_g_I_nominal_value=1  y_g_I_specify=off  y_g_I_priority=None  y_g_I=0  y_g_I_nominal_specify=off  y_g_I_nominal_unit=1  y_g_I_nominal_value=1
      settings: InternalSimscapePortConfiguration="{\"Bottom\":[],\"Left\":[{\"id\":\"A\",\"label\":\"A\",\"type\":\"foundation.moist_air.moist_air\"},{\"id\":\"H\",\"label\":\"H\",\"type\":\"foundation.thermal.thermal\"},{\"id\":\"S\",\"label\":\"S\",\"type\":\"foundation.moist_air.moist_air_source\"}],\"Right\":[{\"id\":\"B\",\"label\":\"B\",\"type\":\"foundation.moist_air.moist_air\"},{\"id\":\"W\",\"label\":\"W\",\"type\":\"output\"},{\"id\":\"F\",\"label\":\"F\",\"type\":\"output\"}],\"Top\":[]}"
  Subsystem4 : Subsystem
  System-Level Heat Exchanger (TL-MA) : SimscapeFluids_lib/Fluid Network Interfaces/Heat Exchangers/System-Level Heat Exchanger (TL-MA)  flow_arrangement=fluids.interfaces.heat_exchangers.enum.SystemLevelFlowArrangementTLMA.Counter  wall_thermal_mass=simscape.enum.onoff.off  mass_wall=1 kg  cp_wall=490 J/(K*kg)  area_A1=.001 m^2  area_B1=.001 m^2  area_A2=.002 m^2  area_B2=.002 m^2  operating_condition_TL=fluids.interfaces.heat_exchangers.enum.SystemLevelOperatingConditionTLMA.Heating  mdot_nominal_TL=0.2 kg/s  delta_p_nominal_TL=0.03 bar  p_in_nominal_TL=1.6 bar  T_in_nominal_TL=20 degC  capacity_spec_TL=fluids.interfaces.heat_exchangers.enum.SystemLevelCapacitySpec.HeatTransfer  Q_nominal=8 kW  T_out_nominal_TL=323.15 K  volume_TL=0.01 m^3  init_spec_TL=fluids.interfaces.heat_exchangers.enum.SystemLevelInitialConditionSpec.Operating  p_init_TL=0.101325 MPa  T_init_TL=293.15 K  mdot_nominal_MA=0.2 kg/s  delta_p_nominal_MA=.05 bar  p_in_nominal_MA=3 bar  T_in_nominal_MA=150 degC  inlet_moisture_spec_MA=foundation.enum.moisture_spec.relative_humidity  RH_in_nominal_MA=0.01  x_w_in_nominal_MA=0.01  y_w_in_nominal_MA=0.01  HR_in_nominal_MA=0.01  inlet_trace_gas_spec_MA=foundation.enum.trace_gas_spec.mass_fraction  x_g_in_nominal_MA=0.001  y_g_in_nominal_MA=0.001  volume_MA=0.005 m^3  init_spec_MA=fluids.interfaces.heat_exchangers.enum.SystemLevelInitialConditionSpec.Operating  p_init_MA=0.101325 MPa  T_init_MA=293.15 K  moisture_spec_MA=foundation.enum.moisture_spec.relative_humidity  RH_init_MA=0.5  x_w_init_MA=0.01  y_w_init_MA=0.01  HR_init_MA=0.01  trace_gas_spec_MA=foundation.enum.trace_gas_spec.mass_fraction  x_g_init_MA=0.001  y_g_init_MA=0.001  RH_ws_MA=1  a_TL=0.023  b_TL=0.8  c_TL=0.33  a_MA=0.023  b_MA=0.8  c_MA=0.33
      settings: InternalSimscapePortConfiguration="{\"Bottom\":[],\"Left\":[{\"id\":\"A1\",\"label\":\"A1\",\"type\":\"foundation.thermal_liquid.thermal_liquid\"},{\"id\":\"B1\",\"label\":\"B1\",\"type\":\"foundation.thermal_liquid.thermal_liquid\"}],\"Right\":[{\"id\":\"A2\",\"label\":\"A2\",\"type\":\"foundation.moist_air.moist_air\"},{\"id\":\"B2\",\"label\":\"B2\",\"type\":\"foundation.moist_air.moist_air\"}],\"Top\":[{\"id\":\"Q1\",\"label\":\"Q1\",\"type\":\"output\"},{\"id\":\"Q2\",\"label\":\"Q2\",\"type\":\"output\"},{\"id\":\"W\",\"label\":\"W\",\"type\":\"output\"}]}"
  Thermal Mass2 : fl_lib/Thermal/Thermal Elements/Thermal Mass  Commented=on  mass_type=foundation.enum.constant_variable.constant  mass=1 kg  sp_heat=910 J/kg/K  mass_min=1e-6 kg  num_ports=foundation.enum.numPorts2.one  m_specify=off  m_priority=High  m=1 kg  m_nominal_specify=off  m_nominal_unit=kg  m_nominal_value=1  T_specify=on  T_priority=High  T=20 degC  T_nominal_specify=off  T_nominal_unit=K  T_nominal_value=1  Q_specify=off  Q_priority=None  Q=0 W  Q_nominal_specify=off  Q_nominal_unit=W  Q_nominal_value=1
  Thermal Reference : fl_lib/Thermal/Thermal Elements/Thermal Reference
  Thermal Reference1 : fl_lib/Thermal/Thermal Elements/Thermal Reference
  Thermal Reference2 : fl_lib/Thermal/Thermal Elements/Thermal Reference
  Throttle valve area curve : fl_lib/Physical Signals/Lookup Tables/PS Lookup Table (1D)  x=[0,.2,.3,.4,.5,.6,.7,.8,.9,1]  f=[0.000011,0.00002,0.00009,0.00020,0.00035,0.00055,0.00077,0.00101,0.00125,0.00153]  interp_method=simscape.enum.interpolation.smooth  extrap_method=simscape.enum.extrapolation.linear
  Throttle valve area curve1 : fl_lib/Physical Signals/Lookup Tables/PS Lookup Table (1D)  x=[0,.2,.3,.4,.5,.6,.7,.8,.9,1]  f=[0.000011,0.00002,0.00009,0.00020,0.00035,0.00055,0.00077,0.00101,0.00125,0.00153]  interp_method=simscape.enum.interpolation.smooth  extrap_method=simscape.enum.extrapolation.linear
  Throttle valve area curve2 : fl_lib/Physical Signals/Lookup Tables/PS Lookup Table (1D)  x=[0,.2,.3,.4,.5,.6,.7,.8,.9,1]  f=[0.0000011,0.000002,0.00009,0.00020,0.00035,0.00055,0.00077,0.00101,0.00125,0.00153]  interp_method=simscape.enum.interpolation.smooth  extrap_method=simscape.enum.extrapolation.linear
  Throttle valve area curve4 : fl_lib/Physical Signals/Lookup Tables/PS Lookup Table (1D)  x=[0,.2,.3,.4,.5,.6,.7,.8,.9,1]  f=[0.0000011,0.000002,0.00009,0.00020,0.00035,0.00055,0.00077,0.00101,0.00125,0.00153]  interp_method=simscape.enum.interpolation.smooth  extrap_method=simscape.enum.extrapolation.linear
  Valve : fl_lib/Moist Air/Elements/Local Restriction (MA)  restriction_type=foundation.enum.restriction_type.variable  restriction_area=0.001 m^2  min_area=2e-5 m^2  max_area=.00165 m^2  area=.002 m^2  Cd=3.5  B_lam=9.44E-01
  Valve1 : fl_lib/Moist Air/Elements/Local Restriction (MA)  restriction_type=foundation.enum.restriction_type.variable  restriction_area=0.001 m^2  min_area=2e-5 m^2  max_area=.00165 m^2  area=.002 m^2  Cd=3.5  B_lam=9.44E-01
  Valve2 : fl_lib/Moist Air/Elements/Local Restriction (MA)  restriction_type=foundation.enum.restriction_type.variable  restriction_area=0.001 m^2  min_area=2e-5 m^2  max_area=.00165 m^2  area=.002 m^2  Cd=3.5  B_lam=9.44E-01
  Valve4 : fl_lib/Moist Air/Elements/Local Restriction (MA)  restriction_type=foundation.enum.restriction_type.variable  restriction_area=0.001 m^2  min_area=2e-5 m^2  max_area=.00165 m^2  area=.002 m^2  Cd=.64  B_lam=9.44E-01
  Valves Closed : fl_lib/Physical Signals/Sources/PS Constant  Commented=on  constant=0
  Valves Open : fl_lib/Physical Signals/Sources/PS Constant  constant=1
  WS removal Rate : fl_lib/Moist Air/Sources/Moisture & Trace Gas Sources/Controlled Moisture Source (MA)  Commented=on  moisture_source_spec=foundation.enum.moisture_source_spec.liquid  Phi_S_specify=off  Phi_S_priority=None  Phi_S=0 kW  Phi_S_nominal_specify=off  Phi_S_nominal_unit=kW  Phi_S_nominal_value=1  mdot_w_S_specify=off  mdot_w_S_priority=None  mdot_w_S=0 kg/s  mdot_w_S_nominal_specify=off  mdot_w_S_nominal_unit=kg/s  mdot_w_S_nominal_value=1
      settings: InternalSimscapePortConfiguration="{\"Bottom\":[],\"Left\":[{\"id\":\"S\",\"label\":\"S\",\"type\":\"foundation.moist_air.moist_air_source\"}],\"Right\":[{\"id\":\"M\",\"label\":\"M\",\"type\":\"input\"},{\"id\":\"T\",\"label\":\"T\",\"type\":\"input\"}],\"Top\":[]}"
  W_add Rate : fl_lib/Moist Air/Sources/Moisture & Trace Gas Sources/Controlled Moisture Source (MA)  moisture_source_spec=foundation.enum.moisture_source_spec.vapor  Phi_S_specify=off  Phi_S_priority=None  Phi_S=0 kW  Phi_S_nominal_specify=off  Phi_S_nominal_unit=kW  Phi_S_nominal_value=1  mdot_w_S_specify=off  mdot_w_S_priority=None  mdot_w_S=0 kg/s  mdot_w_S_nominal_specify=off  mdot_w_S_nominal_unit=kg/s  mdot_w_S_nominal_value=1
      settings: InternalSimscapePortConfiguration="{\"Bottom\":[],\"Left\":[{\"id\":\"S\",\"label\":\"S\",\"type\":\"foundation.moist_air.moist_air_source\"}],\"Right\":[{\"id\":\"M\",\"label\":\"M\",\"type\":\"input\"},{\"id\":\"T\",\"label\":\"T\",\"type\":\"input\"}],\"Top\":[]}"
  s_pos_percent_CHXV_Set : PMIOPort  Side=Left
  CHUdi_T_degC_moisture : PMIOPort  Port=2  Side=Left
  CHUdi_mdot_kg/s_moisture : PMIOPort  Port=3  Side=Left
  CHUwi_mdot_kg/s_moisture : PMIOPort  Port=4  Side=Left
  CHUwi_T_degC_moisture : PMIOPort  Port=5  Side=Left
  CHUdi_RH_%_moisture : PMIOPort  Port=6  Side=Left
  CWS_mdot_kg/s_moisture : PMIOPort  Port=7  Side=Left
  Coolant_from_LT : PMIOPort  Port=8  Side=Right
  Coolant_from_Peripherals : PMIOPort  Port=9  Side=Right
  tag scope: CHX_HR_W=global, CHX_mdot_kgs_water=global, CWS_mdot_kgs_water=global, E_Motor_HR_W=global, FCS_mdot_kgs_water=global, INV_HR_W=global
  wires:
  P_Amb/1 -> Inlet/2(Inport1)
  T_amb/1 -> Inlet/1(Inport)
  s_omega_rpm_EAC_Set/1 -> Simulink-PS Converter4/1
  s_pos_percent_ETV_Set/1 -> Simulink-PS Converter3/1
  PS-Simulink Converter/1 -> [FCS_mdot_kgs_water]
  PS-Simulink Converter1/1 -> [CWS_mdot_kgs_water]
  CHX-Heat-Release/1 -> [CHX_HR_W]
  PS-Simulink Converter2/1 -> [CHX_mdot_kgs_water]
  [LT_INV_HR] -> Simulink-PS Converter8/1
  [LT_EAC_HR] -> Simulink-PS Converter2/1
  INV-Heat-Release/1 -> [INV_HR_W]
  EAC-Heat-Release/1 -> [E_Motor_HR_W]
  [CAx_mdot_water] -> Simulink-PS Converter5/1
  [CAx_Ther_Power] -> Simulink-PS Converter1/1
  [i_Stack] -> Stack2mflowusage/1
  Subsystem4/4(Pressure_LH2) -> Scope/4
  Subsystem4/8(Heat_Evaporator) -> Scope/8
  Stack2mflowusage/1 -> Simulink-PS Converter6/1
  Subsystem4/5(mFlow) -> Scope/5
  Subsystem4/6(mFlow_LH2) -> Scope/6
  Subsystem4/2(Temp_LH2) -> Scope/2
  Subsystem4/7(Heat_FCS) -> Scope/7
  Subsystem4/3(Pressure) -> Scope/3
  Subsystem4/1(Temp- Glysantin) -> Scope/1
  PS-Simulink Converter3/1 -> Gain/1
  Gain/1 -> Scope1/1
  connections:
  Controlled Reservoir (G)1/RConn2 -- Inlet/LConn2
  Controlled Heat Flow Rate Source/RConn2 -- Thermal Reference/LConn1
  S1/LConn1 -- Inlet/RConn1
  Controlled Heat Flow Rate Source/LConn1 -- Stack_Temp/LConn2
  Hydrowell-Exp_VTS/RConn2 -- Mechanical Rotational Reference3/LConn1
  Controlled Reservoir (G)1/RConn1 -- Inlet/LConn1
  Hydrowell_VTS/RConn1 -- S2/LConn1
  Hydrowell_VTS/RConn3 -- Mech Converter/RConn1
  Hydrowell_VTS/LConn1 -- S1/RConn1
  Simulink-PS Converter5/RConn1 -- W_add Rate/RConn1
  Hydrowell_VTS/LConn2 -- Mechanical Rotational Reference1/LConn1
  Stack_Temp/LConn1 -- Valve/RConn1
  Hydrowell_VTS/RConn2 -- Hydrowell-Exp_VTS/LConn2 -- Mech Converter/LConn1
  Mech Converter/RConn2 -- Simulink-PS Converter4/RConn1
  Hydrowell-Exp_VTS/RConn1 -- S8/LConn1
  Controlled Reservoir (G)1/LConn1 -- S8/RConn1
  Valve/LConn2 -- Throttle valve area curve/RConn1
  S4/LConn1 -- Valve/LConn1
  Valve1/LConn2 -- Throttle valve area curve1/RConn1
  Valve1/RConn1 -- S5/LConn1
  Valves Open/RConn1 -- Throttle valve area curve1/LConn1 -- Throttle valve area curve2/LConn1 -- Throttle valve area curve4/LConn1 -- Throttle valve area curve/LConn1
  Valve2/LConn2 -- Throttle valve area curve2/RConn1
  WS removal Rate/LConn1 -- Cond.1/LConn3
  Pipe (MA)2/LConn1 -- S3/LConn1
  Controlled Moisture Source (MA)1/LConn1 -- Pipe (MA)1/LConn3
  Perfect Insulator2/LConn1 -- Pipe (MA)1/LConn2
  Measurement Selector (MA)/LConn1 -- Pipe (MA)1/RConn3
  Controlled Moisture Source (MA)1/RConn2 -- CHUwi_mdot_kg/s_moisture/RConn1
  Measurement Selector (MA)1/LConn1 -- Pipe (MA)2/RConn3
  Perfect Insulator3/LConn1 -- Pipe (MA)2/LConn2
  Controlled Moisture Source (MA)2/LConn1 -- Pipe (MA)2/LConn3
  CHUdi_mdot_kg/s_moisture/RConn1 -- Controlled Moisture Source (MA)2/RConn1
  Controlled Moisture Source (MA)2/RConn2 -- CHUdi_T_degC_moisture/RConn1
  Measurement Selector (MA)1/RConn3 -- CHUdi_RH_%_moisture/RConn1
  CHUwi_T_degC_moisture/RConn1 -- Controlled Moisture Source (MA)1/RConn1
  Valve2/RConn1 -- S6/LConn1
  S5/RConn1 -- Valve2/LConn1
  CWS_mdot_kg/s_moisture/RConn1 -- WS removal Rate/RConn1
  Perfect Insulator1/LConn1 -- Cond.1/LConn2
  Pipe (MA)2/RConn1 -- S4/RConn1
  S6/RConn1 -- Valve4/LConn1
  PS-Simulink Converter/LConn1 -- Stack_Temp/RConn2
  Cond.1/RConn2 -- PS-Simulink Converter1/LConn1
  Hydrowell-Exp_VTS/LConn3 -- Simulink-PS Converter3/RConn1
  Valve4/LConn2 -- Throttle valve area curve4/RConn1
  Valve4/RConn1 -- S7/LConn1
  System-Level Heat Exchanger (TL-MA)/RConn1 -- S3/RConn1
  System-Level Heat Exchanger (TL-MA)/LConn1 -- Flow Rate Sensor (TL)/RConn1
  PS Gain1/RConn1 -- Gate Valve (TL)1/LConn2
  PS-Simulink Converter2/LConn1 -- System-Level Heat Exchanger (TL-MA)/LConn5
  CHX-Heat-Release/LConn1 -- System-Level Heat Exchanger (TL-MA)/LConn3
  Thermal Reference2/LConn1 -- Controlled Heat Flow Rate Source2/RConn2
  Controlled Heat Flow Rate Source2/LConn1 -- Heat Flow Rate Sensor2/LConn1
  Heat Flow Rate Sensor2/RConn2 -- INV/RConn1
  Controlled Heat Flow Rate Source1/LConn1 -- Heat Flow Rate Sensor1/LConn1
  Thermal Reference1/LConn1 -- Controlled Heat Flow Rate Source1/RConn2
  Heat Flow Rate Sensor1/RConn2 -- EAC/RConn1
  Simulink-PS Converter8/RConn1 -- Controlled Heat Flow Rate Source2/RConn1
  Simulink-PS Converter2/RConn1 -- Controlled Heat Flow Rate Source1/RConn1
  Heat Flow Rate Sensor2/RConn1 -- INV-Heat-Release/LConn1
  Heat Flow Rate Sensor1/RConn1 -- EAC-Heat-Release/LConn1
  Simulink-PS Converter1/RConn1 -- Controlled Heat Flow Rate Source/RConn1
  Stack_Temp/RConn1 -- Valve1/LConn1
  W_add Rate/LConn1 -- Stack_Temp/LConn3
  S5/LConn2 -- W_add Rate/RConn2
  S2/RConn1 -- Int. G-MA/LConn1
  System-Level Heat Exchanger (TL-MA)/RConn2 -- Int. G-MA/RConn1
  Int. MA-G/RConn1 -- S7/RConn1
  Hydrowell-Exp_VTS/LConn1 -- Int. MA-G/LConn1
  Sensor LH2 in/LConn1 -- LH2 Properties/RConn1 -- Controlled Mass Flow Rate Source (2P)/RConn1
  Joby Evaporator/LConn4 -- Subsystem4/LConn1
  Reservoir (2P)1/LConn1 -- Sensor LH2 out/RConn1
  Sensor LH2 in/RConn1 -- Joby Evaporator/LConn1
  PS Gain/RConn1 -- Controlled Mass Flow Rate Source (2P)/LConn2
  Sensor LH2 out/LConn1 -- Joby Evaporator/LConn2
  Joby Evaporator/LConn3 -- Subsystem4/LConn2
  Reservoir (2P)2/LConn1 -- Controlled Mass Flow Rate Source (2P)/LConn1
  Simulink-PS Converter6/RConn1 -- PS Gain/LConn1
  Flow Resistance (TL)1/LConn1 -- Coolant_from_Peripherals/RConn1 -- Flow Resistance (TL)1/RConn1 -- Gate Valve (TL)1/LConn1
  Joby Evaporator/RConn2 -- Gate Valve (TL)1/RConn1
  Thermal Mass2/LConn1 -- Environment Temperature4/LConn1 -- Convective Heat Transfer1/RConn1
  Convective Heat Transfer1/LConn1 -- Radiator1/LConn2
  System-Level Heat Exchanger (TL-MA)/LConn2 -- EAC/LConn1
  EAC/LConn2 -- INV/LConn1
  INV/LConn2 -- Coolant_from_LT/RConn1
  Radiator1/LConn1 -- Flow Rate Sensor (TL)/LConn1 -- Radiator1/RConn1 -- Joby Evaporator/RConn1
  Flow Rate Sensor (TL)/RConn3 -- PS-Simulink Converter3/LConn1
  s_pos_percent_CHXV_Set/RConn1 -- PS Gain1/LConn1
